simulink model "StaticThermalAnalysis"  (R2023a)
settings: Solver=VariableStepAuto  StartTime=0.0  StopTime=1.0  RelTol=1e-3
undefined symbols (not defined in the file): Nodes, Settings
libraries: ThermalLibrary x75, fl_lib x28, nesl_utility x15
settings Model: Creator=Lorenzo Capra  LastModifiedBy=Lorenzo Capra

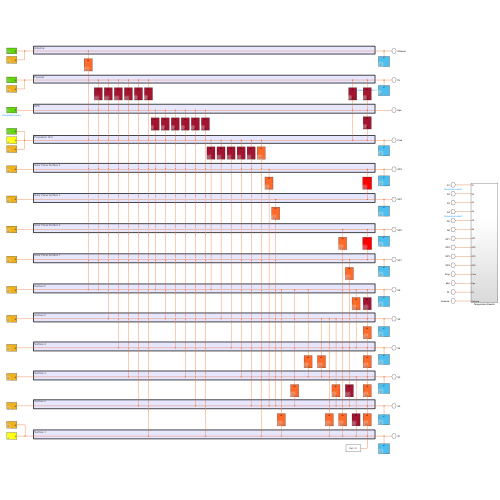
[thumbnail: Simulink's stored preview of the top-level diagram]
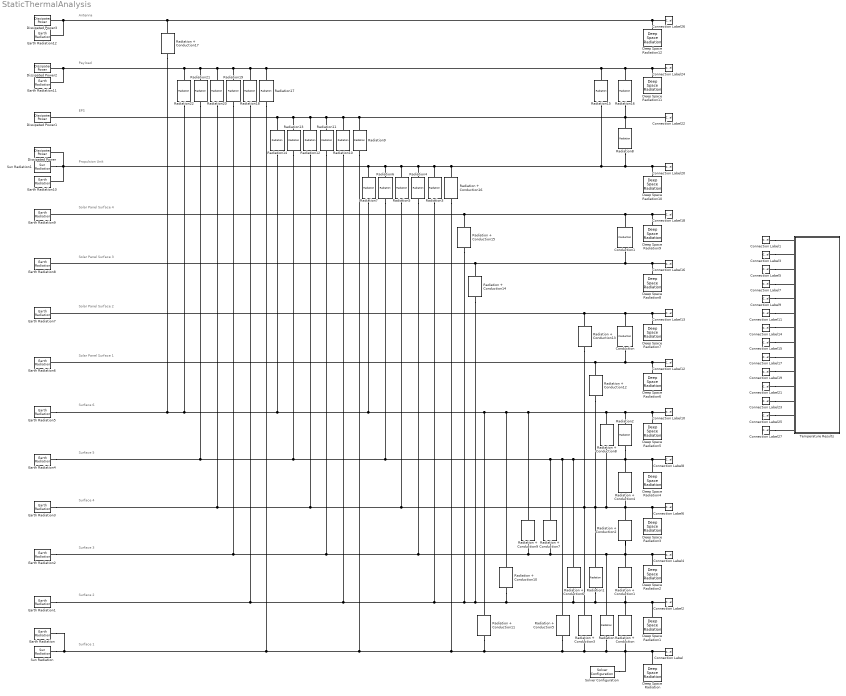
== system StaticThermalAnalysis ==
  note: Surface 1
  note: Surface 2
  note: Surface 3
  note: Surface 4
  note: Surface 5
  note: Surface 6
  note: Solar Panel Surface 1
  note: Solar Panel Surface 2
  note: Solar Panel Surface 3
  note: Solar Panel Surface 4
  note: Propulsion Unit
  note: EPS
  note: Payload
  note: Antenna
  Conduction : ThermalLibrary/Conduction  Ac=Nodes.SP1.Ac  thick1=Nodes.SP1.thickness  conductivity1=Nodes.SP1.conductivity  resistance=Settings.Resistance*0  thick2=Nodes.SP2.thickness  conductivity2=Nodes.SP2.conductivity
  Conduction1 : ThermalLibrary/Conduction  Ac=Nodes.SP3.Ac  thick1=Nodes.SP3.thickness  conductivity1=Nodes.SP3.conductivity  resistance=Settings.Resistance*0  thick2=Nodes.SP4.thickness  conductivity2=Nodes.SP4.conductivity
  Connection Label : ConnectionLabel  Label=S1
  Connection Label1 : ConnectionLabel  Label=S1
  Connection Label10 : ConnectionLabel  Label=S6
  Connection Label11 : ConnectionLabel  Label=S6
  Connection Label12 : ConnectionLabel  Label=SP1
  Connection Label13 : ConnectionLabel  Label=SP2
  Connection Label14 : ConnectionLabel  Label=SP1
  Connection Label15 : ConnectionLabel  Label=SP2
  Connection Label16 : ConnectionLabel  Label=SP3
  Connection Label17 : ConnectionLabel  Label=SP3
  Connection Label18 : ConnectionLabel  Label=SP4
  Connection Label19 : ConnectionLabel  Label=SP4
  Connection Label2 : ConnectionLabel  Label=S2
  Connection Label20 : ConnectionLabel  Label=Prop
  Connection Label21 : ConnectionLabel  Label=Prop
  Connection Label22 : ConnectionLabel  Label=Eps
  Connection Label23 : ConnectionLabel  Label=Eps
  Connection Label24 : ConnectionLabel  Label=PL
  Connection Label25 : ConnectionLabel  Label=PL
  Connection Label26 : ConnectionLabel  Label=Antenna
  Connection Label27 : ConnectionLabel  Label=Antenna
  Connection Label3 : ConnectionLabel  Label=S2
  Connection Label4 : ConnectionLabel  Label=S3
  Connection Label5 : ConnectionLabel  Label=S3
  Connection Label6 : ConnectionLabel  Label=S4
  Connection Label7 : ConnectionLabel  Label=S4
  Connection Label8 : ConnectionLabel  Label=S5
  Connection Label9 : ConnectionLabel  Label=S5
  Deep Space Radiation : ThermalLibrary/Deep Space Radiation  T_deep_space=Settings.T_deep_space  A=Nodes.S1.A  emissivity=Nodes.S1.emissivity
  Deep Space Radiation1 : ThermalLibrary/Deep Space Radiation  T_deep_space=Settings.T_deep_space  A=Nodes.S2.A  emissivity=Nodes.S2.emissivity
  Deep Space Radiation10 : ThermalLibrary/Deep Space Radiation  T_deep_space=Settings.T_deep_space  A=Nodes.Prop.A  emissivity=Nodes.Prop.emissivity
  Deep Space Radiation11 : ThermalLibrary/Deep Space Radiation  T_deep_space=Settings.T_deep_space  A=Nodes.PL.A  emissivity=Nodes.PL.emissivity
  Deep Space Radiation12 : ThermalLibrary/Deep Space Radiation  T_deep_space=Settings.T_deep_space  A=Nodes.Antenna.A  emissivity=Nodes.Antenna.emissivity
  Deep Space Radiation2 : ThermalLibrary/Deep Space Radiation  T_deep_space=Settings.T_deep_space  A=Nodes.S3.A  emissivity=Nodes.S3.emissivity
  Deep Space Radiation3 : ThermalLibrary/Deep Space Radiation  T_deep_space=Settings.T_deep_space  A=Nodes.S4.A  emissivity=Nodes.S4.emissivity
  Deep Space Radiation4 : ThermalLibrary/Deep Space Radiation  T_deep_space=Settings.T_deep_space  A=Nodes.S5.A  emissivity=Nodes.S5.emissivity
  Deep Space Radiation5 : ThermalLibrary/Deep Space Radiation  T_deep_space=Settings.T_deep_space  A=Nodes.S6.A  emissivity=Nodes.S6.emissivity
  Deep Space Radiation6 : ThermalLibrary/Deep Space Radiation  T_deep_space=Settings.T_deep_space  A=Nodes.SP1.A  emissivity=Nodes.SP1.emissivity
  Deep Space Radiation7 : ThermalLibrary/Deep Space Radiation  T_deep_space=Settings.T_deep_space  A=Nodes.SP1.A  emissivity=Nodes.SP1.emissivity
  Deep Space Radiation8 : ThermalLibrary/Deep Space Radiation  T_deep_space=Settings.T_deep_space  A=Nodes.SP3.A  emissivity=Nodes.SP3.emissivity
  Deep Space Radiation9 : ThermalLibrary/Deep Space Radiation  T_deep_space=Settings.T_deep_space  A=Nodes.SP4.A  emissivity=Nodes.SP4.emissivity
  Dissipated Power : ThermalLibrary/Dissipated Power  Pdiss=Nodes.Prop.Pdiss
  Dissipated Power1 : ThermalLibrary/Dissipated Power  Pdiss=Nodes.Eps.Pdiss
  Dissipated Power2 : ThermalLibrary/Dissipated Power  Pdiss=Nodes.PL.Pdiss
  Dissipated Power3 : ThermalLibrary/Dissipated Power  Pdiss=Nodes.Antenna.Pdiss
  Earth Radiation : ThermalLibrary/Earth Radiation  T_earth=Settings.T_earth  A=Nodes.S1.A  emissivity=Nodes.S1.emissivity  alfa=Nodes.S1.alfa
  Earth Radiation1 : ThermalLibrary/Earth Radiation  T_earth=Settings.T_earth  A=Nodes.S2.A  emissivity=Nodes.S2.emissivity  alfa=Nodes.S2.alfa
  Earth Radiation10 : ThermalLibrary/Earth Radiation  T_earth=Settings.T_earth  A=Nodes.Prop.A  emissivity=Nodes.Prop.emissivity  alfa=Nodes.Prop.alfa
  Earth Radiation11 : ThermalLibrary/Earth Radiation  T_earth=Settings.T_earth  A=Nodes.PL.A  emissivity=Nodes.PL.emissivity  alfa=Nodes.PL.alfa
  Earth Radiation12 : ThermalLibrary/Earth Radiation  T_earth=Settings.T_earth  A=Nodes.Antenna.A  emissivity=Nodes.Antenna.emissivity  alfa=Nodes.Antenna.alfa
  Earth Radiation2 : ThermalLibrary/Earth Radiation  T_earth=Settings.T_earth  A=Nodes.S3.A  emissivity=Nodes.S3.emissivity  alfa=Nodes.S3.alfa
  Earth Radiation3 : ThermalLibrary/Earth Radiation  T_earth=Settings.T_earth  A=Nodes.S4.A  emissivity=Nodes.S4.emissivity  alfa=Nodes.S4.alfa
  Earth Radiation4 : ThermalLibrary/Earth Radiation  T_earth=Settings.T_earth  A=Nodes.S5.A  emissivity=Nodes.S5.emissivity  alfa=Nodes.S5.alfa
  Earth Radiation5 : ThermalLibrary/Earth Radiation  T_earth=Settings.T_earth  A=Nodes.S6.A  emissivity=Nodes.S6.emissivity  alfa=Nodes.S6.alfa
  Earth Radiation6 : ThermalLibrary/Earth Radiation  T_earth=Settings.T_earth  A=Nodes.SP1.A  emissivity=Nodes.SP1.emissivity  alfa=Nodes.SP1.alfa
  Earth Radiation7 : ThermalLibrary/Earth Radiation  T_earth=Settings.T_earth  A=Nodes.SP2.A  emissivity=Nodes.SP2.emissivity  alfa=Nodes.SP2.alfa
  Earth Radiation8 : ThermalLibrary/Earth Radiation  T_earth=Settings.T_earth  A=Nodes.SP3.A  emissivity=Nodes.SP3.emissivity  alfa=Nodes.SP3.alfa
  Earth Radiation9 : ThermalLibrary/Earth Radiation  T_earth=Settings.T_earth  A=Nodes.SP4.A  emissivity=Nodes.SP4.emissivity  alfa=Nodes.SP4.alfa
  Radiation : ThermalLibrary/Radiation  A1=Nodes.S1.A  emissivity1=Nodes.S1.emissivity  F12=Nodes.S1.F  A2=Nodes.S3.A  emissivity2=Nodes.S3.emissivity  F21=Nodes.S3.F
  Radiation + Conduction : ThermalLibrary/Radiation + Conduction  A1=Nodes.S1.A  emissivity1=Nodes.S1.emissivity  F12=Nodes.S1.F  A2=Nodes.S2.A  emissivity2=Nodes.S2.emissivity  F21=Nodes.S2.F  Ac=Nodes.S1.Ac  thick1=Nodes.S1.thickness  conductivity1=Nodes.S1.conductivity  resistance=Settings.Resistance  thick2=Nodes.S2.thickness  conductivity2=Nodes.S2.conductivity
  Radiation + Conduction1 : ThermalLibrary/Radiation + Conduction  A1=Nodes.S2.A  emissivity1=Nodes.S2.emissivity  F12=Nodes.S2.F  A2=Nodes.S3.A  emissivity2=Nodes.S3.emissivity  F21=Nodes.S3.F  Ac=Nodes.S2.Ac  thick1=Nodes.S2.thickness  conductivity1=Nodes.S2.conductivity  resistance=Settings.Resistance  thick2=Nodes.S3.thickness  conductivity2=Nodes.S3.conductivity
  Radiation + Conduction10 : ThermalLibrary/Radiation + Conduction  A1=Nodes.S2.A  emissivity1=Nodes.S2.emissivity  F12=Nodes.S2.F  A2=Nodes.S6.A  emissivity2=Nodes.S6.emissivity  F21=Nodes.S6.F  Ac=Nodes.S2.Ac  thick1=Nodes.S2.thickness  conductivity1=Nodes.S2.conductivity  resistance=Settings.Resistance  thick2=Nodes.S6.thickness  conductivity2=Nodes.S6.conductivity
  Radiation + Conduction11 : ThermalLibrary/Radiation + Conduction  A1=Nodes.S1.A  emissivity1=Nodes.S1.emissivity  F12=Nodes.S1.F  A2=Nodes.S6.A  emissivity2=Nodes.S6.emissivity  F21=Nodes.S6.F  Ac=Nodes.S1.Ac  thick1=Nodes.S1.thickness  conductivity1=Nodes.S1.conductivity  resistance=Settings.Resistance  thick2=Nodes.S6.thickness  conductivity2=Nodes.S6.conductivity
  Radiation + Conduction12 : ThermalLibrary/Radiation + Conduction  A1=Nodes.S4.A  emissivity1=Nodes.S4.emissivity  F12=Nodes.S4.F  A2=Nodes.SP1.A  emissivity2=Nodes.SP1.emissivity  F21=Nodes.SP1.F  Ac=Nodes.S4.Ac  thick1=Nodes.S4.thickness  conductivity1=Nodes.S4.conductivity  resistance=Settings.Resistance  thick2=Nodes.SP1.thickness  conductivity2=Nodes.SP1.conductivity
  Radiation + Conduction13 : ThermalLibrary/Radiation + Conduction  A1=Nodes.S4.A  emissivity1=Nodes.S4.emissivity  F12=Nodes.S4.F  A2=Nodes.SP2.A  emissivity2=Nodes.SP2.emissivity  F21=Nodes.SP2.F  Ac=Nodes.S4.Ac  thick1=Nodes.S4.thickness  conductivity1=Nodes.S4.conductivity  resistance=Settings.Resistance  thick2=Nodes.SP2.thickness  conductivity2=Nodes.SP2.conductivity
  Radiation + Conduction14 : ThermalLibrary/Radiation + Conduction  A1=Nodes.S2.A  emissivity1=Nodes.S2.emissivity  F12=Nodes.S2.F  A2=Nodes.SP3.A  emissivity2=Nodes.SP3.emissivity  F21=Nodes.SP3.F  Ac=Nodes.S2.Ac  thick1=Nodes.S2.thickness  conductivity1=Nodes.S2.conductivity  resistance=Settings.Resistance  thick2=Nodes.SP3.thickness  conductivity2=Nodes.SP3.conductivity
  Radiation + Conduction15 : ThermalLibrary/Radiation + Conduction  A1=Nodes.S2.A  emissivity1=Nodes.S2.emissivity  F12=Nodes.S2.F  A2=Nodes.SP4.A  emissivity2=Nodes.SP4.emissivity  F21=Nodes.SP4.F  Ac=Nodes.S2.Ac  thick1=Nodes.S2.thickness  conductivity1=Nodes.S2.conductivity  resistance=Settings.Resistance  thick2=Nodes.SP4.thickness  conductivity2=Nodes.SP4.conductivity
  Radiation + Conduction16 : ThermalLibrary/Radiation + Conduction  A1=Nodes.S1.A  emissivity1=Nodes.S1.emissivity  F12=Nodes.S1.F  A2=Nodes.Prop.A  emissivity2=Nodes.Prop.emissivity  F21=Nodes.Prop.F  Ac=Nodes.S1.Ac  thick1=Nodes.S1.thickness  conductivity1=Nodes.S1.conductivity  resistance=Settings.Resistance  thick2=Nodes.Prop.thickness  conductivity2=Nodes.Prop.conductivity
  Radiation + Conduction17 : ThermalLibrary/Radiation + Conduction  A1=Nodes.S6.A  emissivity1=Nodes.S6.emissivity  F12=Nodes.S6.F  A2=Nodes.Antenna.A  emissivity2=Nodes.Antenna.emissivity  F21=Nodes.Antenna.F  Ac=Nodes.S6.Ac  thick1=Nodes.S6.thickness  conductivity1=Nodes.S6.conductivity  resistance=Settings.Resistance  thick2=Nodes.Antenna.thickness  conductivity2=Nodes.Antenna.conductivity
  Radiation + Conduction2 : ThermalLibrary/Radiation + Conduction  A1=Nodes.S3.A  emissivity1=Nodes.S3.emissivity  F12=Nodes.S3.F  A2=Nodes.S4.A  emissivity2=Nodes.S4.emissivity  F21=Nodes.S4.F  Ac=Nodes.S3.Ac  thick1=Nodes.S3.thickness  conductivity1=Nodes.S3.conductivity  resistance=Settings.Resistance  thick2=Nodes.S4.thickness  conductivity2=Nodes.S4.conductivity
  Radiation + Conduction3 : ThermalLibrary/Radiation + Conduction  A1=Nodes.S1.A  emissivity1=Nodes.S1.emissivity  F12=Nodes.S1.F  A2=Nodes.S4.A  emissivity2=Nodes.S4.emissivity  F21=Nodes.S4.F  Ac=Nodes.S1.Ac  thick1=Nodes.S1.thickness  conductivity1=Nodes.S1.conductivity  resistance=Settings.Resistance  thick2=Nodes.S4.thickness  conductivity2=Nodes.S4.conductivity
  Radiation + Conduction4 : ThermalLibrary/Radiation + Conduction  A1=Nodes.S4.A  emissivity1=Nodes.S4.emissivity  F12=Nodes.S4.F  A2=Nodes.S5.A  emissivity2=Nodes.S5.emissivity  F21=Nodes.S5.F  Ac=Nodes.S4.Ac  thick1=Nodes.S4.thickness  conductivity1=Nodes.S4.conductivity  resistance=Settings.Resistance  thick2=Nodes.S5.thickness  conductivity2=Nodes.S5.conductivity
  Radiation + Conduction5 : ThermalLibrary/Radiation + Conduction  A1=Nodes.S1.A  emissivity1=Nodes.S1.emissivity  F12=Nodes.S1.F  A2=Nodes.S5.A  emissivity2=Nodes.S5.emissivity  F21=Nodes.S5.F  Ac=Nodes.S1.Ac  thick1=Nodes.S1.thickness  conductivity1=Nodes.S1.conductivity  resistance=Settings.Resistance  thick2=Nodes.S5.thickness  conductivity2=Nodes.S5.conductivity
  Radiation + Conduction6 : ThermalLibrary/Radiation + Conduction  A1=Nodes.S2.A  emissivity1=Nodes.S2.emissivity  F12=Nodes.S2.F  A2=Nodes.S5.A  emissivity2=Nodes.S5.emissivity  F21=Nodes.S5.F  Ac=Nodes.S2.Ac  thick1=Nodes.S2.thickness  conductivity1=Nodes.S2.conductivity  resistance=Settings.Resistance  thick2=Nodes.S5.thickness  conductivity2=Nodes.S5.conductivity
  Radiation + Conduction7 : ThermalLibrary/Radiation + Conduction  A1=Nodes.S3.A  emissivity1=Nodes.S3.emissivity  F12=Nodes.S3.F  A2=Nodes.S5.A  emissivity2=Nodes.S5.emissivity  F21=Nodes.S5.F  Ac=Nodes.S3.Ac  thick1=Nodes.S3.thickness  conductivity1=Nodes.S3.conductivity  resistance=Settings.Resistance  thick2=Nodes.S5.thickness  conductivity2=Nodes.S5.conductivity
  Radiation + Conduction8 : ThermalLibrary/Radiation + Conduction  A1=Nodes.S4.A  emissivity1=Nodes.S4.emissivity  F12=Nodes.S4.F  A2=Nodes.S6.A  emissivity2=Nodes.S6.emissivity  F21=Nodes.S6.F  Ac=Nodes.S4.Ac  thick1=Nodes.S4.thickness  conductivity1=Nodes.S4.conductivity  resistance=Settings.Resistance  thick2=Nodes.S6.thickness  conductivity2=Nodes.S6.conductivity
  Radiation + Conduction9 : ThermalLibrary/Radiation + Conduction  A1=Nodes.S3.A  emissivity1=Nodes.S3.emissivity  F12=Nodes.S3.F  A2=Nodes.S6.A  emissivity2=Nodes.S6.emissivity  F21=Nodes.S6.F  Ac=Nodes.S3.Ac  thick1=Nodes.S3.thickness  conductivity1=Nodes.S3.conductivity  resistance=Settings.Resistance  thick2=Nodes.S6.thickness  conductivity2=Nodes.S6.conductivity
  Radiation1 : ThermalLibrary/Radiation  A1=Nodes.S2.A  emissivity1=Nodes.S2.emissivity  F12=Nodes.S2.F  A2=Nodes.S4.A  emissivity2=Nodes.S4.emissivity  F21=Nodes.S4.F
  Radiation10 : ThermalLibrary/Radiation  A1=Nodes.S2.A  emissivity1=Nodes.S2.emissivity  F12=Nodes.S2.F  A2=Nodes.Eps.A  emissivity2=Nodes.Eps.emissivity  F21=Nodes.Eps.F
  Radiation11 : ThermalLibrary/Radiation  A1=Nodes.S3.A  emissivity1=Nodes.S3.emissivity  F12=Nodes.S3.F  A2=Nodes.Eps.A  emissivity2=Nodes.Eps.emissivity  F21=Nodes.Eps.F
  Radiation12 : ThermalLibrary/Radiation  A1=Nodes.S4.A  emissivity1=Nodes.S4.emissivity  F12=Nodes.S4.F  A2=Nodes.Eps.A  emissivity2=Nodes.Eps.emissivity  F21=Nodes.Eps.F
  Radiation13 : ThermalLibrary/Radiation  A1=Nodes.S5.A  emissivity1=Nodes.S5.emissivity  F12=Nodes.S5.F  A2=Nodes.Eps.A  emissivity2=Nodes.Eps.emissivity  F21=Nodes.Eps.F
  Radiation14 : ThermalLibrary/Radiation  A1=Nodes.S6.A  emissivity1=Nodes.S6.emissivity  F12=Nodes.S6.F  A2=Nodes.Eps.A  emissivity2=Nodes.Eps.emissivity  F21=Nodes.Eps.F
  Radiation15 : ThermalLibrary/Radiation  A1=Nodes.Prop.A  emissivity1=Nodes.Prop.emissivity  F12=Nodes.Prop.F  A2=Nodes.PL.A  emissivity2=Nodes.PL.emissivity  F21=Nodes.PL.F
  Radiation16 : ThermalLibrary/Radiation  A1=Nodes.Eps.A  emissivity1=Nodes.Eps.emissivity  F12=Nodes.Eps.F  A2=Nodes.PL.A  emissivity2=Nodes.PL.emissivity  F21=Nodes.PL.F
  Radiation17 : ThermalLibrary/Radiation  A1=Nodes.S1.A  emissivity1=Nodes.S1.emissivity  F12=Nodes.S1.F  A2=Nodes.PL.A  emissivity2=Nodes.PL.emissivity  F21=Nodes.PL.F
  Radiation18 : ThermalLibrary/Radiation  A1=Nodes.S2.A  emissivity1=Nodes.S2.emissivity  F12=Nodes.S2.F  A2=Nodes.PL.A  emissivity2=Nodes.PL.emissivity  F21=Nodes.PL.F
  Radiation19 : ThermalLibrary/Radiation  A1=Nodes.S3.A  emissivity1=Nodes.S3.emissivity  F12=Nodes.S3.F  A2=Nodes.PL.A  emissivity2=Nodes.PL.emissivity  F21=Nodes.PL.F
  Radiation2 : ThermalLibrary/Radiation  A1=Nodes.S5.A  emissivity1=Nodes.S5.emissivity  F12=Nodes.S5.F  A2=Nodes.S6.A  emissivity2=Nodes.S6.emissivity  F21=Nodes.S6.F
  Radiation20 : ThermalLibrary/Radiation  A1=Nodes.S4.A  emissivity1=Nodes.S4.emissivity  F12=Nodes.S4.F  A2=Nodes.PL.A  emissivity2=Nodes.PL.emissivity  F21=Nodes.PL.F
  Radiation21 : ThermalLibrary/Radiation  A1=Nodes.S5.A  emissivity1=Nodes.S5.emissivity  F12=Nodes.S5.F  A2=Nodes.PL.A  emissivity2=Nodes.PL.emissivity  F21=Nodes.PL.F
  Radiation22 : ThermalLibrary/Radiation  A1=Nodes.S6.A  emissivity1=Nodes.S6.emissivity  F12=Nodes.S6.F  A2=Nodes.PL.A  emissivity2=Nodes.PL.emissivity  F21=Nodes.PL.F
  Radiation3 : ThermalLibrary/Radiation  A1=Nodes.S2.A  emissivity1=Nodes.S2.emissivity  F12=Nodes.S2.F  A2=Nodes.Prop.A  emissivity2=Nodes.Prop.emissivity  F21=Nodes.Prop.F
  Radiation4 : ThermalLibrary/Radiation  A1=Nodes.S3.A  emissivity1=Nodes.S3.emissivity  F12=Nodes.S3.F  A2=Nodes.Prop.A  emissivity2=Nodes.Prop.emissivity  F21=Nodes.Prop.F
  Radiation5 : ThermalLibrary/Radiation  A1=Nodes.S4.A  emissivity1=Nodes.S4.emissivity  F12=Nodes.S4.F  A2=Nodes.Prop.A  emissivity2=Nodes.Prop.emissivity  F21=Nodes.Prop.F
  Radiation6 : ThermalLibrary/Radiation  A1=Nodes.S5.A  emissivity1=Nodes.S5.emissivity  F12=Nodes.S5.F  A2=Nodes.Prop.A  emissivity2=Nodes.Prop.emissivity  F21=Nodes.Prop.F
  Radiation7 : ThermalLibrary/Radiation  A1=Nodes.S6.A  emissivity1=Nodes.S6.emissivity  F12=Nodes.S6.F  A2=Nodes.Prop.A  emissivity2=Nodes.Prop.emissivity  F21=Nodes.Prop.F
  Radiation8 : ThermalLibrary/Radiation  A1=Nodes.Prop.A  emissivity1=Nodes.Prop.emissivity  F12=Nodes.Prop.F  A2=Nodes.Eps.A  emissivity2=Nodes.Eps.emissivity  F21=Nodes.Eps.F
  Radiation9 : ThermalLibrary/Radiation  A1=Nodes.S1.A  emissivity1=Nodes.S1.emissivity  F12=Nodes.S1.F  A2=Nodes.Eps.A  emissivity2=Nodes.Eps.emissivity  F21=Nodes.Eps.F
  Solver Configuration : nesl_utility/Solver Configuration  PhysicalDomain=network_engine_domain  SubClassName=solver  LeftPortType=input  RightPortType=generic  Tones=[]  Harmonics=[]  SimulateNoise=off  Profile=off  UseLocalSampling=off  EnableSwitchedLinearOptims=on  FrequencyDomain=off  UseCCode=off  RelTol=0.001  AbsTol=0.001  MinStep=1e-09  ToWorkspace=off  RevertToSquareIcSolve=off  NumHomotopyIterations=100  PhasorMode=off  PhasorModeNumHarmonics=1  ConsistencySolver=NEWTON_XTOL_AFTER_FTOL  IndexReductionMethod=DerivativeReplacement  DoDC=off  ResidualTolerance=1e-09  ConsistencyTolSource=GLOBAL  ConsistencyAbsTol=0.001  ConsistencyRelTol=0.001  ConsistencyTolFactor=0.001  UseLocalSolver=off  LocalSolverChoice=NE_BACKWARD_EULER_ADVANCER  ResolveIndetEquations=on  FunctionEvalNumThread=1  LocalSolverSampleTime=0.001  DoFixedCost=off  MaxNonlinIter=3  MaxModeIter=2  ComputeImpulses=off  ImpulseIterations=2  LinearAlgebra=auto  LinearAlgebraNumThread=0  EquationFormulation=NE_TIME_EF  DelaysMemoryBudget=1024  AutomaticFiltering=on  FilteringTimeConstant=0.001  PartitionStorageMethod=AS_NEEDED  PartitionMemoryBudget=1024  PartitionMethod=ROBUST
  Sun Radiation : ThermalLibrary/Sun Radiation  A=Nodes.S1.A  alfa=Nodes.S1.alfa
  Sun Radiation1 : ThermalLibrary/Sun Radiation  A=Nodes.Prop.A  alfa=Nodes.Prop.alfa
  Temperature Results : Subsystem
  connections:
  Deep Space Radiation/RConn1 -- Connection Label/LConn1 -- Solver Configuration/RConn1 -- Radiation + Conduction/LConn1 -- Radiation/LConn1 -- Radiation + Conduction3/LConn1 -- Radiation + Conduction5/LConn1 -- Sun Radiation/RConn1 -- Earth Radiation/RConn1 -- Radiation17/LConn1 -- Radiation9/LConn1 -- Radiation + Conduction16/LConn1 -- Radiation + Conduction11/LConn1
  Connection Label1/LConn1 -- Temperature Results/LConn1
  Connection Label3/LConn1 -- Temperature Results/LConn2
  Connection Label5/LConn1 -- Temperature Results/LConn3
  Earth Radiation3/RConn1 -- Radiation20/LConn1 -- Radiation12/LConn1 -- Radiation5/LConn1 -- Radiation + Conduction13/LConn1 -- Radiation + Conduction3/RConn1 -- Radiation + Conduction12/LConn1 -- Radiation1/RConn1 -- Radiation + Conduction8/LConn1 -- Deep Space Radiation3/RConn1 -- Connection Label6/LConn1 -- Radiation + Conduction4/LConn1 -- Radiation + Conduction2/RConn1
  Deep Space Radiation1/RConn1 -- Connection Label2/LConn1 -- Radiation1/LConn1 -- Radiation + Conduction6/LConn1 -- Earth Radiation1/RConn1 -- Radiation18/LConn1 -- Radiation10/LConn1 -- Radiation3/LConn1 -- Radiation + Conduction15/LConn1 -- Radiation + Conduction14/LConn1 -- Radiation + Conduction10/LConn1 -- Radiation + Conduction1/LConn1 -- Radiation + Conduction/RConn1
  Connection Label7/LConn1 -- Temperature Results/LConn4
  Connection Label8/LConn1 -- Deep Space Radiation4/RConn1 -- Radiation2/LConn1 -- Earth Radiation4/RConn1 -- Radiation21/LConn1 -- Radiation13/LConn1 -- Radiation6/LConn1 -- Radiation + Conduction7/RConn1 -- Radiation + Conduction5/RConn1 -- Radiation + Conduction6/RConn1 -- Radiation + Conduction4/RConn1
  Connection Label9/LConn1 -- Temperature Results/LConn5
  Connection Label10/LConn1 -- Deep Space Radiation5/RConn1 -- Earth Radiation5/RConn1 -- Radiation + Conduction17/LConn1 -- Radiation22/LConn1 -- Radiation14/LConn1 -- Radiation7/LConn1 -- Radiation + Conduction11/RConn1 -- Radiation + Conduction10/RConn1 -- Radiation + Conduction9/RConn1 -- Radiation + Conduction8/RConn1 -- Radiation2/RConn1
  Radiation + Conduction2/LConn1 -- Earth Radiation2/RConn1 -- Radiation19/LConn1 -- Radiation11/LConn1 -- Radiation4/LConn1 -- Radiation + Conduction9/LConn1 -- Radiation + Conduction7/LConn1 -- Radiation/RConn1 -- Radiation + Conduction1/RConn1 -- Deep Space Radiation2/RConn1 -- Connection Label4/LConn1
  Connection Label11/LConn1 -- Temperature Results/LConn6
  Connection Label12/LConn1 -- Deep Space Radiation6/RConn1 -- Radiation + Conduction12/RConn1 -- Earth Radiation6/RConn1 -- Conduction/LConn1
  Deep Space Radiation7/RConn1 -- Radiation + Conduction13/RConn1 -- Earth Radiation7/RConn1 -- Conduction/RConn1 -- Connection Label13/LConn1
  Connection Label14/LConn1 -- Temperature Results/LConn7
  Connection Label15/LConn1 -- Temperature Results/LConn8
  Deep Space Radiation8/RConn1 -- Radiation + Conduction14/RConn1 -- Earth Radiation8/RConn1 -- Conduction1/LConn1 -- Connection Label16/LConn1
  Connection Label17/LConn1 -- Temperature Results/LConn9
  Earth Radiation9/RConn1 -- Radiation + Conduction15/RConn1 -- Conduction1/RConn1 -- Deep Space Radiation9/RConn1 -- Connection Label18/LConn1
  Connection Label19/LConn1 -- Temperature Results/LConn10
  Deep Space Radiation10/RConn1 -- Connection Label20/LConn1 -- Radiation8/LConn1 -- Radiation15/LConn1 -- Radiation + Conduction16/RConn1 -- Radiation4/RConn1 -- Radiation5/RConn1 -- Radiation6/RConn1 -- Radiation7/RConn1 -- Earth Radiation10/RConn1 -- Dissipated Power/RConn1 -- Sun Radiation1/RConn1 -- Radiation3/RConn1
  Connection Label21/LConn1 -- Temperature Results/LConn11
  Connection Label22/LConn1 -- Radiation16/LConn1 -- Radiation8/RConn1 -- Radiation9/RConn1 -- Radiation10/RConn1 -- Radiation11/RConn1 -- Radiation12/RConn1 -- Radiation14/RConn1 -- Dissipated Power1/RConn1 -- Radiation13/RConn1
  Connection Label23/LConn1 -- Temperature Results/LConn12
  Connection Label24/LConn1 -- Deep Space Radiation11/RConn1 -- Radiation16/RConn1 -- Radiation15/RConn1 -- Radiation17/RConn1 -- Radiation18/RConn1 -- Radiation19/RConn1 -- Radiation20/RConn1 -- Radiation21/RConn1 -- Radiation22/RConn1 -- Dissipated Power2/RConn1 -- Earth Radiation11/RConn1
  Connection Label25/LConn1 -- Temperature Results/LConn13
  Deep Space Radiation12/RConn1 -- Radiation + Conduction17/RConn1 -- Earth Radiation12/RConn1 -- Dissipated Power3/RConn1 -- Connection Label26/LConn1
  Connection Label27/LConn1 -- Temperature Results/LConn14

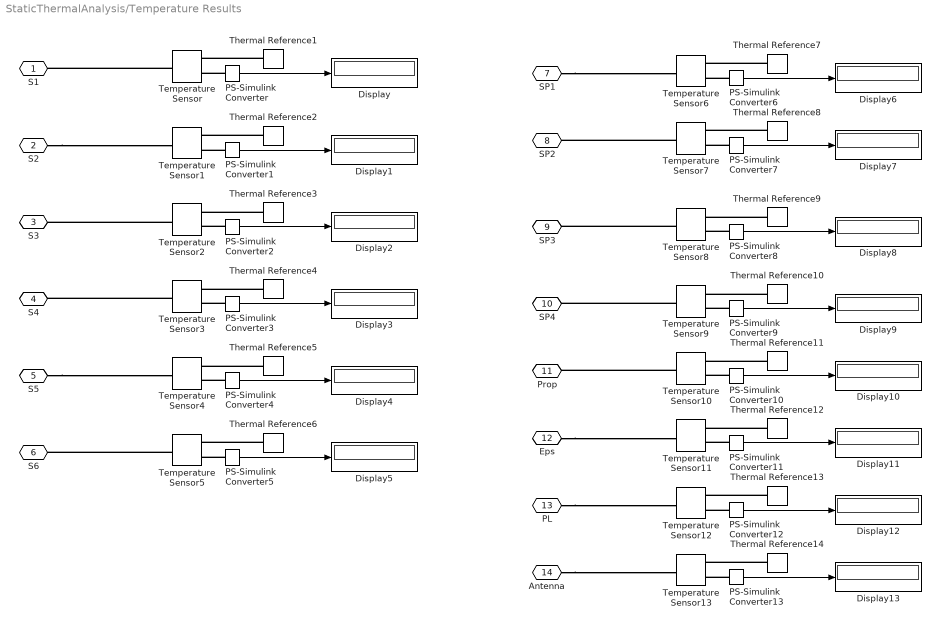
== system StaticThermalAnalysis/Temperature Results ==
  Display{,1..13} (14 alike) : Display
  PS-Simulink Converter{,1..13} (14 alike) : nesl_utility/PS-Simulink Converter  PhysicalDomain=network_engine_domain  SubClassName=ps_output  LeftPortType=input  RightPortType=output  PseudoPeriodic=off  Frequencies=[]  VectorFormat=inherit  Unit=inherit  AffineConversion=off
  Temperature Sensor{,1..13} (14 alike) : fl_lib/Thermal/Thermal Sensors/Temperature Sensor  temperature_measure=foundation.enum.MeasurementReference.difference
  Thermal Reference{1..14} (14 alike) : fl_lib/Thermal/Thermal Elements/Thermal Reference
  S1 : PMIOPort  Side=Left
  S2 : PMIOPort  Port=2  Side=Left
  S3 : PMIOPort  Port=3  Side=Left
  S4 : PMIOPort  Port=4  Side=Left
  S5 : PMIOPort  Port=5  Side=Left
  S6 : PMIOPort  Port=6  Side=Left
  SP1 : PMIOPort  Port=7  Side=Left
  SP2 : PMIOPort  Port=8  Side=Left
  SP3 : PMIOPort  Port=9  Side=Left
  SP4 : PMIOPort  Port=10  Side=Left
  Prop : PMIOPort  Port=11  Side=Left
  Eps : PMIOPort  Port=12  Side=Left
  PL : PMIOPort  Port=13  Side=Left
  Antenna : PMIOPort  Port=14  Side=Left
  wires:
  PS-Simulink Converter/1 -> Display/1
  PS-Simulink Converter1/1 -> Display1/1
  PS-Simulink Converter2/1 -> Display2/1
  PS-Simulink Converter3/1 -> Display3/1
  PS-Simulink Converter4/1 -> Display4/1
  PS-Simulink Converter5/1 -> Display5/1
  PS-Simulink Converter6/1 -> Display6/1
  PS-Simulink Converter7/1 -> Display7/1
  PS-Simulink Converter8/1 -> Display8/1
  PS-Simulink Converter9/1 -> Display9/1
  PS-Simulink Converter10/1 -> Display10/1
  PS-Simulink Converter11/1 -> Display11/1
  PS-Simulink Converter12/1 -> Display12/1
  PS-Simulink Converter13/1 -> Display13/1
  connections:
  PS-Simulink Converter/LConn1 -- Temperature Sensor/RConn2
  Thermal Reference1/LConn1 -- Temperature Sensor/RConn1
  Temperature Sensor/LConn1 -- S1/RConn1
  PS-Simulink Converter1/LConn1 -- Temperature Sensor1/RConn2
  Thermal Reference2/LConn1 -- Temperature Sensor1/RConn1
  S2/RConn1 -- Temperature Sensor1/LConn1
  Temperature Sensor2/LConn1 -- S3/RConn1
  Thermal Reference3/LConn1 -- Temperature Sensor2/RConn1
  PS-Simulink Converter2/LConn1 -- Temperature Sensor2/RConn2
  Thermal Reference4/LConn1 -- Temperature Sensor3/RConn1
  Temperature Sensor3/LConn1 -- S4/RConn1
  PS-Simulink Converter3/LConn1 -- Temperature Sensor3/RConn2
  Thermal Reference5/LConn1 -- Temperature Sensor4/RConn1
  S5/RConn1 -- Temperature Sensor4/LConn1
  PS-Simulink Converter4/LConn1 -- Temperature Sensor4/RConn2
  PS-Simulink Converter5/LConn1 -- Temperature Sensor5/RConn2
  Thermal Reference6/LConn1 -- Temperature Sensor5/RConn1
  Temperature Sensor5/LConn1 -- S6/RConn1
  PS-Simulink Converter6/LConn1 -- Temperature Sensor6/RConn2
  SP1/RConn1 -- Temperature Sensor6/LConn1
  Thermal Reference7/LConn1 -- Temperature Sensor6/RConn1
  Temperature Sensor7/LConn1 -- SP2/RConn1
  Thermal Reference8/LConn1 -- Temperature Sensor7/RConn1
  PS-Simulink Converter7/LConn1 -- Temperature Sensor7/RConn2
  Temperature Sensor8/LConn1 -- SP3/RConn1
  Thermal Reference9/LConn1 -- Temperature Sensor8/RConn1
  PS-Simulink Converter8/LConn1 -- Temperature Sensor8/RConn2
  PS-Simulink Converter9/LConn1 -- Temperature Sensor9/RConn2
  Thermal Reference10/LConn1 -- Temperature Sensor9/RConn1
  Temperature Sensor9/LConn1 -- SP4/RConn1
  Temperature Sensor10/LConn1 -- Prop/RConn1
  Thermal Reference11/LConn1 -- Temperature Sensor10/RConn1
  PS-Simulink Converter10/LConn1 -- Temperature Sensor10/RConn2
  PS-Simulink Converter11/LConn1 -- Temperature Sensor11/RConn2
  Eps/RConn1 -- Temperature Sensor11/LConn1
  Thermal Reference12/LConn1 -- Temperature Sensor11/RConn1
  PL/RConn1 -- Temperature Sensor12/LConn1
  Thermal Reference13/LConn1 -- Temperature Sensor12/RConn1
  PS-Simulink Converter12/LConn1 -- Temperature Sensor12/RConn2
  Antenna/RConn1 -- Temperature Sensor13/LConn1
  Thermal Reference14/LConn1 -- Temperature Sensor13/RConn1
  PS-Simulink Converter13/LConn1 -- Temperature Sensor13/RConn2
